simulink model "WaterTankModel_SimpleScenario"  (Simulink 8.1)
settings: Solver=ode3  StartTime=0.0  StopTime=180.0  FixedStep=0.001  RelTol=1e-3
InitFcn:
  | initparametersDACADC
undefined symbols (not defined in the file): Ad, Bd, Cd, Dd, x0
libraries: GisooLib x3
settings Model: Creator=behdad  LastModifiedBy=behdad

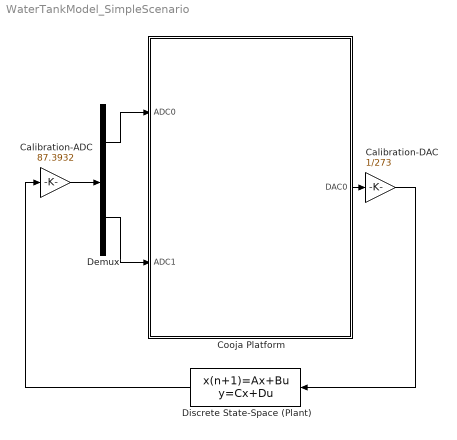
== system WaterTankModel_SimpleScenario ==
  Calibration-ADC : Gain  Gain=87.3932
  Calibration-DAC : Gain  Gain=1/273
  Cooja Platform : Subsystem  AncestorBlock=GisooLib/Gisoo Platform  TreatAsAtomicUnit=on
  Demux : Demux  Outputs=2
  Discrete State-Space (Plant) : DiscreteStateSpace  A=Ad  B=Bd  C=Cd  D=Dd  X0=x0  SampleTime=-1
  wires:
  Discrete State-Space (Plant)/1 -> Calibration-ADC/1
  Calibration-ADC/1 -> Demux/1
  Demux/1 -> Cooja Platform/1(ADC0)
  Demux/2 -> Cooja Platform/2(ADC1)
  Calibration-DAC/1 -> Discrete State-Space (Plant)/1
  Cooja Platform/1(DAC0) -> Calibration-DAC/1

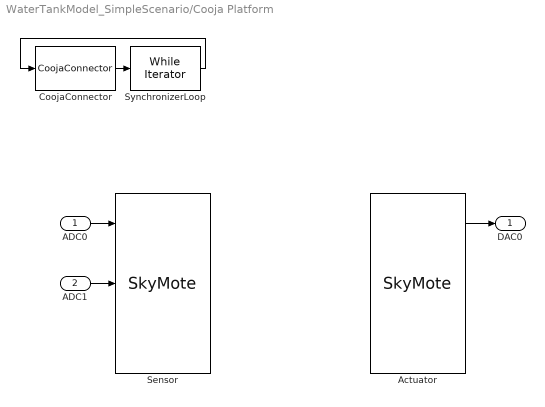
== system WaterTankModel_SimpleScenario/Cooja Platform ==
  ADC0 : Inport
  ADC1 : Inport  Port=2
  Actuator : GisooLib/SkyMote  moteID=4  PacketType=6
  CoojaConnector : GisooLib/Cooja Platform/CoojaConnector
  Sensor : GisooLib/SkyMote  moteID=1  PacketType=6
  SynchronizerLoop : WhileIterator  MaxIters=-1  WhileBlockType=do-while  ShowIterationPort=on
  DAC0 : Outport
  wires:
  Actuator/1 -> DAC0/1
  ADC0/1 -> Sensor/1
  ADC1/1 -> Sensor/2
  SynchronizerLoop/1 -> CoojaConnector/1
  CoojaConnector/1 -> SynchronizerLoop/1
